simulink model "Test_Encoder_8_to_3"  (R2023a)
settings: Solver=ode45  StartTime=0.0  StopTime=len  RelTol=1e-3  EnableMultiTasking=on
libraries: simulink x2, Encoders_Lib x1
settings Model: Creator=N  LastModifiedBy=Jozko Mrkvicka
settings SolverCC: AlgebraicLoopSolver=TrustRegion
settings DataIOCC: SaveFormat=Array  ReturnWorkspaceOutputs=off
settings OptimizationCC: LifeSpan=inf
settings DebuggingCC: UnconnectedInputMsg=warning  UnconnectedOutputMsg=warning  UnconnectedLineMsg=warning  SFUnexpectedBacktrackingDiag=warning  SFNoUnconditionalDefaultTransitionDiag=warning  ArithmeticOperatorsInVariantConditions=warning
settings HardwareCC: ProdWordSize=32
settings ModelReferenceCC: EnableRefExpFcnMdlSchedulingChecks=on
settings SFSimCC: SimUseLocalCustomCode=off  CustomCodeUndefinedFunction=UseInterfaceOnly
settings RTWCC: RTWUseLocalCustomCode=off
settings CodeAppCC: StateflowObjectComments=on
settings GRTTargetCC: TargetLangStandard=C89/C90 (ANSI)
settings ConfigComp: CovMetricSettings=dw  CovSaveCumulativeToWorkspaceVar=on  CovSaveSingleToWorkspaceVar=on  CovExternalEMLEnable=off

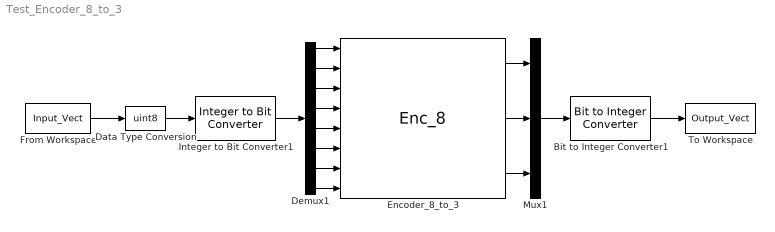
== system Test_Encoder_8_to_3 ==
  Bit to Integer Converter1 : simulink/Logic and Bit Operations/Bit to Integer Converter  nbits=3  bitOrder=MSB first  signedOutputValues=Unsigned  outDtype=uint8  outDtypeSigned=Inherit via internal rule
      settings: LibrarySourceBlock=|
      | commutil2/Bit to Integer
      | Converter
  Data Type Conversion : DataTypeConversion  OutDataTypeStr=uint8  SaturateOnIntegerOverflow=off  RndMeth=Floor
  Demux1 : Demux  Outputs=8
  Encoder_8_to_3 : Encoders_Lib/Enc_8  SystemSampleTime=-1  VariantActivationTime=update diagram  Latency=0  AutoFrameSizeCalculation=off
  From Workspace : FromWorkspace  VariableName=Input_Vect  SampleTime=1  Interpolate=off  ZeroCross=off  OutputAfterFinalValue=Holding final value
  Integer to Bit Converter1 : simulink/Logic and Bit Operations/Integer to Bit Converter  nbits=8  signedInputValues=Unsigned  bitOrder=MSB first  outDtype=boolean
      settings: LibrarySourceBlock=|
      | commutil2/Integer to Bit
      | Converter
  Mux1 : Mux  Inputs=3
  To Workspace : ToWorkspace  VariableName=Output_Vect  SampleTime=1
  wires:
  Integer to Bit Converter1/1 -> Demux1/1
  Demux1/1 -> Encoder_8_to_3/1
  Demux1/2 -> Encoder_8_to_3/2
  Demux1/3 -> Encoder_8_to_3/3
  Demux1/4 -> Encoder_8_to_3/4
  Demux1/5 -> Encoder_8_to_3/5
  Demux1/6 -> Encoder_8_to_3/6
  Demux1/7 -> Encoder_8_to_3/7
  Demux1/8 -> Encoder_8_to_3/8
  Mux1/1 -> Bit to Integer Converter1/1
  Encoder_8_to_3/2 -> Mux1/2
  Encoder_8_to_3/1 -> Mux1/1
  Encoder_8_to_3/3 -> Mux1/3
  Data Type Conversion/1 -> Integer to Bit Converter1/1
  Bit to Integer Converter1/1 -> To Workspace/1
  From Workspace/1 -> Data Type Conversion/1
